simulink model "AERO421_FP7"  (R2024b)
settings: Solver=ode3  StartTime=0.0  StopTime=tspan  FixedStep=5  RelTol=1e-3
values from neighbouring files (symbols this model uses):
  E_b_ECI_0 = C2EulerAngles(C_b_ECI_0)    [AERO421_FP7_RJFSR.m]
  I_s = diag([1.2, 1.2, 1.2])    [AERO421_FP7_RJFSR.m]
  J = J + I_w1 + I_w2 + I_w3    [AERO421_FP7_RJFSR.m]
  JD_0 = 2460390    [AERO421_FP7_RJFSR.m]
  Kd = J*eye(3)*2*zeta*wn    [AERO421_FP7_RJFSR.m]
  Kp = 2*J*eye(3)*wn^2    [AERO421_FP7_RJFSR.m]
  m_b = [0; 0; -0.5]    [AERO421_FP7_RJFSR.m]
  max_T = 1    [AERO421_FP7_RJFSR.m]
  q_b_ECI_0 = rotm2quat(C_b_ECI_0)    [AERO421_FP7_RJFSR.m]
  sun_ECI = [0 0 -1]    [AERO421_FP7_RJFSR.m]
  surfaceProperties = [Areas cps normals ... (first row only)    [AERO421_FP7_RJFSR.m]
  w_b_ECI_0 = [0.001; -0.001; 0.002]    [AERO421_FP7_RJFSR.m]
undefined symbols (not defined in the file or in its folder): r_ECI_0, v_ECI_0
libraries: aerolibutil x1
settings Model: Creator=rosha  LastModifiedBy=rosha

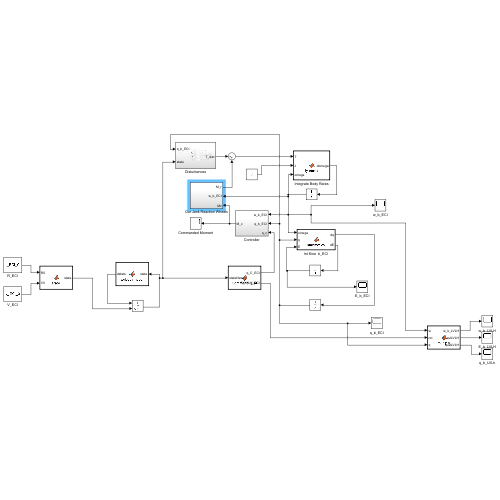
[thumbnail: Simulink's stored preview of the top-level diagram]
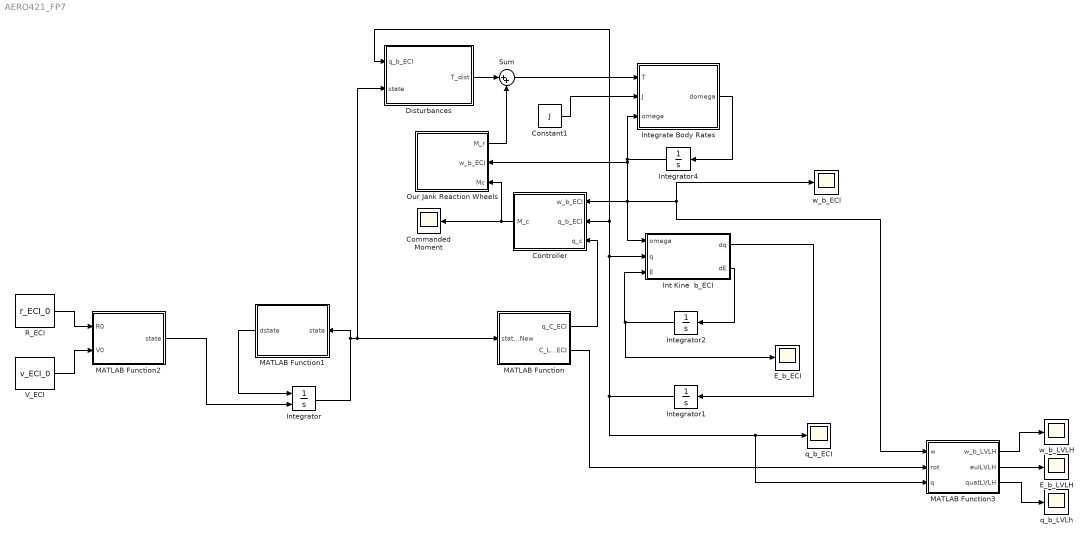
== system AERO421_FP7 ==
  Commanded Moment : Scope
  Constant1 : Constant  Value=J
  Controller : Subsystem
  Disturbances : Subsystem
  E_b_ECI : Scope
  E_b_LVLH : Scope
  Int Kine  b_ECI : MATLAB Function  TreatAsAtomicUnit=on
  Integrate Body Rates : MATLAB Function  TreatAsAtomicUnit=on
  Integrator : Integrator  InitialConditionSource=external
  Integrator1 : Integrator  InitialCondition=q_b_ECI_0
  Integrator2 : Integrator  InitialCondition=E_b_ECI_0
  Integrator4 : Integrator  InitialCondition=w_b_ECI_0
  MATLAB Function : MATLAB Function  TreatAsAtomicUnit=on
  MATLAB Function1 : MATLAB Function  TreatAsAtomicUnit=on
  MATLAB Function2 : MATLAB Function  TreatAsAtomicUnit=on
  MATLAB Function3 : MATLAB Function  TreatAsAtomicUnit=on
  Our Jank Reaction Wheels : Subsystem
      settings: PortSchema="{\"entries\":[{\"content\":{\"sides\":[{\"content\":{\"connectorIds\":[\"Out1\",\"In1\",\"In2\"]},\"type\":\"ConnectorPlacement.EquallySpacedRectSide\",\"uuid\":\"c07e65a8-3a09-4163-ab9e-2228d2e52ec5\"},{\"content\":{\"side\":\"RIGHT\"},\"type\":\"ConnectorPlacement.EquallySpacedRectSide\",\"uuid\":\"64fc0568-6df4-40c5-97b1-a675a03b9b7b\"},{\"content\":{\"side\":\"TOP\"},\"type\":\"ConnectorPlacement.EquallySpacedRectSide\",\"uuid\":\"6ced51b5-350f-46bd-bff5-546870cdfb70\"}]},\"type\":\"ConnectorPlacement.EquallySpacedConnector\",\"uuid\":\"a6912720-308f-478a-9475-f02870833daa\"}],\"packageUris\":[\"http://schema.mathworks.com/mf0/Connector/R2020b\"],\"version\":\"1.0\"}"
  R_ECI : Constant  Value=r_ECI_0
  Sum : Sum  Inputs=|++
  V_ECI : Constant  Value=v_ECI_0
  q_b_ECI : Scope
  q_b_LVLh : Scope
  w_b_ECI : Scope
  w_b_LVLH : Scope
  wires:
  Integrator1/1 -> Disturbances/1(q_b_ECI), Controller/2(q_b_ECI), Int Kine  b_ECI/2(q), MATLAB Function3/3(q), q_b_ECI/1
  MATLAB Function3/2(eulLVLH) -> E_b_LVLH/1
  Constant1/1 -> Integrate Body Rates/2(J)
  V_ECI/1 -> MATLAB Function2/2(V0)
  Integrator2/1 -> E_b_ECI/1, Int Kine  b_ECI/3(E)
  MATLAB Function3/1(w_b_LVLH) -> w_b_LVLH/1
  MATLAB Function/1(q_C_ECI) -> Controller/3(q_c)
  MATLAB Function2/1(state) -> Integrator/2
  MATLAB Function/2(C_LVLH_ECI) -> MATLAB Function3/2(rot)
  Int Kine  b_ECI/2(dE) -> Integrator2/1
  Controller/1(M_c) -> Commanded Moment/1, Our Jank Reaction Wheels/2(Mc)
  Our Jank Reaction Wheels/1(M_r) -> Sum/2
  Integrate Body Rates/1(domega) -> Integrator4/1
  Int Kine  b_ECI/1(dq) -> Integrator1/1
  Integrator4/1 -> Our Jank Reaction Wheels/1(w_b_ECI), MATLAB Function3/1(w), w_b_ECI/1, Int Kine  b_ECI/1(omega), Controller/1(w_b_ECI), Integrate Body Rates/3(omega)
  R_ECI/1 -> MATLAB Function2/1(R0)
  MATLAB Function1/1(dstate) -> Integrator/1
  MATLAB Function3/3(quatLVLH) -> q_b_LVLh/1
  Integrator/1 -> Disturbances/2(state), MATLAB Function/1(stateNew), MATLAB Function1/1(state)
  Disturbances/1(T_dist) -> Sum/1
  Sum/1 -> Integrate Body Rates/1(T)

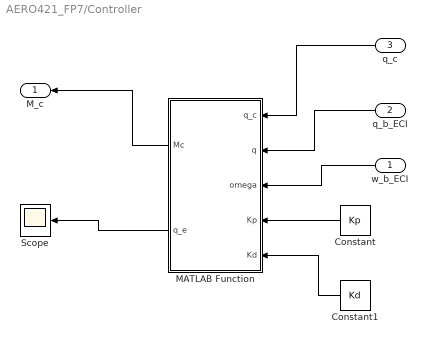
== system AERO421_FP7/Controller ==
  w_b_ECI : Inport  PortDimensions=[3 1]
  q_b_ECI : Inport  Port=2  PortDimensions=[4 1]
  q_c : Inport  Port=3  PortDimensions=[4 1]
  Constant : Constant  Value=Kp
  Constant1 : Constant  Value=Kd
  MATLAB Function : MATLAB Function  TreatAsAtomicUnit=on
  Scope : Scope
  M_c : Outport  PortDimensions=[3 1]  VectorParamsAs1DForOutWhenUnconnected=off
  wires:
  MATLAB Function/1(Mc) -> M_c/1
  q_c/1 -> MATLAB Function/1(q_c)
  q_b_ECI/1 -> MATLAB Function/2(q)
  w_b_ECI/1 -> MATLAB Function/3(omega)
  Constant/1 -> MATLAB Function/4(Kp)
  Constant1/1 -> MATLAB Function/5(Kd)
  MATLAB Function/2(q_e) -> Scope/1

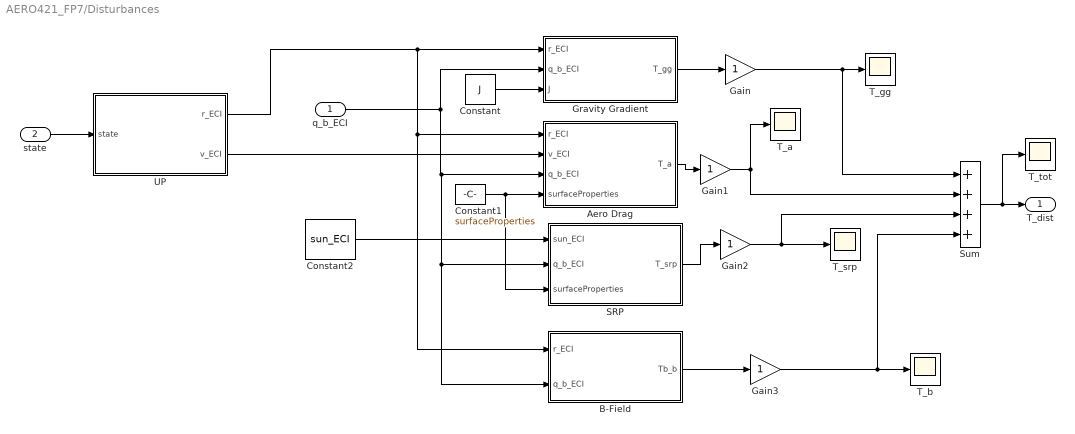
== system AERO421_FP7/Disturbances ==
  q_b_ECI : Inport
  state : Inport  Port=2
  Aero Drag : MATLAB Function  TreatAsAtomicUnit=on
  B-Field : Subsystem
  Constant : Constant  Value=J
  Constant1 : Constant  Value=surfaceProperties
  Constant2 : Constant  Value=sun_ECI
  Gain{,1..3} (4 alike) : Gain
  Gravity Gradient : MATLAB Function  TreatAsAtomicUnit=on
  SRP : MATLAB Function  TreatAsAtomicUnit=on
  Sum : Sum  Inputs=++++
  T_a : Scope
  T_b : Scope
  T_gg : Scope
  T_srp : Scope
  T_tot : Scope
  UP : MATLAB Function  TreatAsAtomicUnit=on
  T_dist : Outport
  wires:
  Sum/1 -> T_tot/1, T_dist/1
  Aero Drag/1(T_a) -> Gain1/1
  Gravity Gradient/1(T_gg) -> Gain/1
  SRP/1(T_srp) -> Gain2/1
  Constant1/1 -> SRP/3(surfaceProperties), Aero Drag/4(surfaceProperties)
  UP/2(v_ECI) -> Aero Drag/2(v_ECI)
  q_b_ECI/1 -> B-Field/2(q_b_ECI), SRP/2(q_b_ECI), Aero Drag/3(q_b_ECI), Gravity Gradient/2(q_b_ECI)
  Constant/1 -> Gravity Gradient/3(J)
  Constant2/1 -> SRP/1(sun_ECI)
  UP/1(r_ECI) -> B-Field/1(r_ECI), Aero Drag/1(r_ECI), Gravity Gradient/1(r_ECI)
  B-Field/1(Tb_b) -> Gain3/1
  Gain/1 -> Sum/1, T_gg/1
  Gain1/1 -> Sum/2, T_a/1
  Gain2/1 -> Sum/3, T_srp/1
  Gain3/1 -> T_b/1, Sum/4
  state/1 -> UP/1(state)

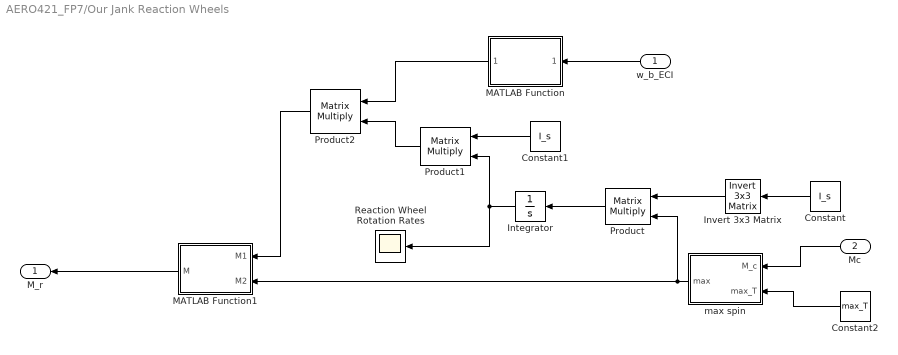
== system AERO421_FP7/Our Jank Reaction Wheels ==
  w_b_ECI : Inport  PortDimensions=[3 1]
  Mc : Inport  Port=2
  Constant : Constant  Value=I_s
  Constant1 : Constant  Value=I_s
  Constant2 : Constant  Value=max_T
  Integrator : Integrator
  Invert 3x3 Matrix : aerolibutil/Invert  3x3 Matrix
  MATLAB Function : MATLAB Function  TreatAsAtomicUnit=on
  MATLAB Function1 : MATLAB Function  TreatAsAtomicUnit=on
  Product : Product  Multiplication=Matrix(*)
  Product1 : Product  Multiplication=Matrix(*)
  Product2 : Product  Multiplication=Matrix(*)
  Reaction Wheel Rotation Rates : Scope
  max spin : MATLAB Function  TreatAsAtomicUnit=on
  M_r : Outport  PortDimensions=[3 1]  VectorParamsAs1DForOutWhenUnconnected=off
  wires:
  MATLAB Function1/1(M) -> M_r/1
  w_b_ECI/1 -> MATLAB Function/1(omega)
  Invert 3x3 Matrix/1 -> Product/1
  Constant/1 -> Invert 3x3 Matrix/1
  Product/1 -> Integrator/1
  Integrator/1 -> Reaction Wheel Rotation Rates/1, Product1/2
  Constant1/1 -> Product1/1
  Product2/1 -> MATLAB Function1/1(M1)
  Product1/1 -> Product2/2
  MATLAB Function/1(omegaX) -> Product2/1
  max spin/1(max) -> Product/2, MATLAB Function1/2(M2)
  Mc/1 -> max spin/1(M_c)
  Constant2/1 -> max spin/2(max_T)

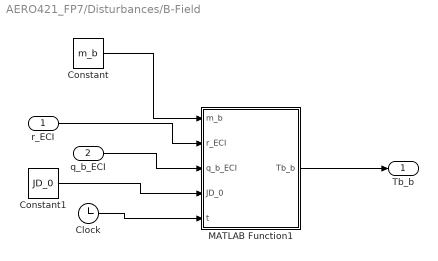
== system AERO421_FP7/Disturbances/B-Field ==
  r_ECI : Inport
  q_b_ECI : Inport  Port=2
  Clock : Clock
  Constant : Constant  Value=m_b  VectorParams1D=off
  Constant1 : Constant  Value=JD_0
  MATLAB Function1 : MATLAB Function  TreatAsAtomicUnit=on
  Tb_b : Outport
  wires:
  MATLAB Function1/1(Tb_b) -> Tb_b/1
  q_b_ECI/1 -> MATLAB Function1/3(q_b_ECI)
  r_ECI/1 -> MATLAB Function1/2(r_ECI)
  Clock/1 -> MATLAB Function1/5(t)
  Constant1/1 -> MATLAB Function1/4(JD_0)
  Constant/1 -> MATLAB Function1/1(m_b)

== matlab function AERO421_FP7/Disturbances/Gravity Gradient ==
  data: r_ECI input; T_gg output; q_b_ECI input; J input
function T_gg = gg_torque(r_ECI, q_b_ECI, J)
mu = 398600; % km^3/s^2

C_b_ECI = quat2dcm(q_b_ECI');
r_b = C_b_ECI * r_ECI;

T_gg = 3*mu/norm(r_ECI)^5*vcross(r_b)*J*r_b;

end

== matlab function AERO421_FP7/Controller/MATLAB Function ==
  data: q_c input; Mc output; q input; omega input; Kp input; Kd input; q_e output
function [Mc,q_e]  = control_law(q_c, q, omega, Kp, Kd)
%#codegen

%q_e = quatMult(quatConjugate(q_c), q);
q_e = quatMult(q, quatConjugate(q_c));
Mc = -Kp*q_e(1:3,1) - Kd*omega;

== matlab function AERO421_FP7/Disturbances/SRP ==
  data: sun_ECI input; T_srp output; q_b_ECI input; surfaceProperties input
function T_srp  = SPR_torque(sun_ECI, q_b_ECI, surfaceProperties)

p_sun = 4.5e-6; %N/m (given)
C_b_ECI_0 = quat2dcm(q_b_ECI');
sun_b = C_b_ECI_0*sun_ECI;
sun_hat = sun_b/norm(sun_b);
T_srp = [0; 0; 0];

for i = 1:length(surfaceProperties)
    % Find wetted area
    normVect = surfaceProperties(i, 5:7);
    normVect = normVect/norm(normVect);
    cpa = surfaceProperties(i, 2:4);
    areaSurf = surfaceProperties(i, 1);
    A_wet = areaSurf*dot(normVect, sun_hat);
    if A_wet > 0
        % Add to total torque from solar pressure
        F_sun = -p_sun*sun_hat*A_wet;
        T_srp = T_srp + cross(cpa', F_sun);
    end
end
end

== matlab function AERO421_FP7/Disturbances/UP ==
  data: state input; r_ECI output; v_ECI output
function [r_ECI, v_ECI]  = unpack(state)

r_ECI = state(1:3)';
v_ECI = state(4:6)';

== matlab function AERO421_FP7/Our Jank Reaction Wheels/max spin ==
  data: M_c input; max output; max_T input
function max = maxT(M_c,max_T)

if norm(M_c) <= max_T
    max = M_c;
else
    max = max_T * M_c/norm(M_c);
end

== matlab function AERO421_FP7/Our Jank Reaction Wheels/MATLAB Function1 ==
  data: M1 input; M output; M2 input
function M = matAdd(M1, M2)
M = M1 + M2;

== matlab function AERO421_FP7/Our Jank Reaction Wheels/MATLAB Function ==
  data: omega input; omegaX output
function omegaX = omegaCross(omega)
omegaX = vcross(omega);

== matlab function AERO421_FP7/MATLAB Function ==
  data: stateNew input; q_C_ECI output; C_LVLH_ECI output
function [q_C_ECI,C_LVLH_ECI] = CommandQuat(stateNew)

R = [stateNew(end,1); stateNew(end,2); stateNew(end,3)];
V = [stateNew(end,4); stateNew(end,5); stateNew(end,6)];

R = R'; %in ECI
V = V';

Z_lvlh = -R/norm(R);
Y_lvlh = -cross(R,V)/norm(cross(R,V));
X_lvlh = cross(Y_lvlh,Z_lvlh);

C_LVLH_ECI = [X_lvlh',Y_lvlh',Z_lvlh'];
C_ECI_LVLH = C_LVLH_ECI';

pointingLVLH = [0;0;-1]; %pointing nadir (always at ground station)

eul = C_ECI_LVLH*pointingLVLH;

q = eul2quat(eul')';
n = q(1);
e = q(2:4);

q_C_ECI = [e;n];

== matlab function AERO421_FP7/MATLAB Function1 ==
  data: state input; dstate output
function dstate = twobodymotion(state) %dstate is derivitve of state
%FUNCTION put in descrip    

mu = 398600;

    %define vars
    x = state(1);
    y = state(2);
    z = state(3);
    dx = state(4); %vel
    dy = state(5); %vel
    dz = state(6); %vel
    
    %mag of pos vector
    r = norm([x y z]);
    
    %accel: !!eqs of motion!!
    ddx = -mu*x/r^3;
    ddy = -mu*y/r^3;
    ddz = -mu*z/r^3;
    
    dstate = [dx; dy; dz; ddx; ddy; ddz]';

end

== matlab function AERO421_FP7/Int Kine  b_ECI ==
  data: omega input; q input; dq output; E input; dE output
function [dq,dE] = kinematics(omega, q, E)
%#codegen

% unpack quaternion

epsilon = q(1:3,1);
eta = q(4,1);

depsilon = 1/2*(eta*eye(3) + vcross(epsilon))*omega;
deta = -1/2*epsilon'*omega;

dq = [depsilon; deta];

LBI = 1/cos(E(2))*[cos(E(2)) sin(E(1))*sin(E(2))  cos(E(1))*sin(E(2));
                   0         cos(E(1))*cos(E(2)) -sin(E(1))*cos(E(2));
                   0         sin(E(1))            cos(E(1))];

dE = LBI*omega;

== matlab function AERO421_FP7/Integrate Body Rates ==
  data: T input; J input; omega input; domega output
function domega = dynamics(T, J, omega)
%#codegen

domega = J\(T - cross(omega, J*omega));

== matlab function AERO421_FP7/MATLAB Function2 ==
  data: R0 input; state output; V0 input
function state = state(R0,V0)

state = [R0',V0'];

== matlab function AERO421_FP7/MATLAB Function3 ==
  data: w input; rot input; w_b_LVLH output; q input; eulLVLH output; quatLVLH output
function [w_b_LVLH,eulLVLH,quatLVLH] = multiply(w,rot,q)

w_b_LVLH = rot*w;

n = q(4);
e = q(1:3)';
quat = [n,e];
eul = quat2eul(quat);

eulLVLH = rot*eul';

q2 = eul2quat(eulLVLH')';
n = q2(1);
e = q2(2:4);
quatLVLH = [e;n];

== matlab function AERO421_FP7/Disturbances/Aero Drag ==
  data: r_ECI input; v_ECI input; T_a output; q_b_ECI input; surfaceProperties input
function T_a = aero_drag_torque(r_ECI, v_ECI, q_b_ECI, surfaceProperties) 
r_ECI = r_ECI*1000; % m
v_ECI = v_ECI*1000; % m/s
% Convert v_ECI to v_b
C_b_ECI_0 = quat2dcm(q_b_ECI');
v_b = C_b_ECI_0*v_ECI;
v_hat = v_b/norm(v_b);
% Calculate density using standard exponetial decay model (or model of your
% choice)
Re = 6378*1000;
Me = 5.972e+24;
h = norm(r_ECI) - Re;
G = 6.67e-11;
k = 1.381e-23;
rho0 = 3.614e-14;
Cd = 2.2;

g = G*Me/norm(r_ECI)^2;

m = 28.964/6.022e23; % CHECK UNITS
T = - 131.21 + 0.00299*h;
H = 109*1000;
h0 = 700*1000;
rho = rho0*exp(-((h-h0)/H));
T_a = [0; 0; 0];
% P = 22.65 * exp(1.73 - .000157 * h);
% rho = P/(0.2869*(T+273.15));



% Loop through all the surfaces of the MehielSat
for i = 1:length(surfaceProperties)
    % Find wetted area
    normVect = surfaceProperties(i, 5:7);
    normVect = normVect/norm(normVect);
    cpa = surfaceProperties(i, 2:4);
    areaSurf = surfaceProperties(i, 1);
    A_wet = areaSurf*dot(normVect, v_hat);
    if A_wet > 0
        % Add to total torque from atmospheric drag
        Fdrag = -0.5*Cd*rho*norm(v_b)^2*A_wet*v_hat;
        T_a = T_a + cross(cpa', Fdrag);
    end


end

== matlab function AERO421_FP7/Disturbances/B-Field/MATLAB Function1 ==
  data: m_b input; r_ECI input; q_b_ECI input; Tb_b output; JD_0 input; t input
function Tb_b = WMM(m_b, r_ECI, q_b_ECI, JD_0, t)

% Constants
omega_Earth = 7.2921150e-5; % Earth's rotation rate in rad/s
r_ECI = r_ECI*1000; %convert to meters

% Time since JD_0 (in days)
delta_JD = t / 86400; % 86400 sec/day

% Current Julian Date
JD = JD_0 + delta_JD;
pos = omega_Earth*JD;
r_ECEF = rotz(rad2deg(pos))' * r_ECI;

C_b_ECI = quat2dcm(q_b_ECI');
C_ECI_ECEF = rotz(rad2deg(pos));
C_b_ECEF = C_b_ECI * C_ECI_ECEF;

% DGRF 2020 (given)
a = 6371.2; %km
g_11 = -1450.9; %nT
h_11 = 4652.5; %nT
g_10 = -29404.8; %nT
m_ECEF = a^3*[g_11; h_11; g_10]; %nT km^3
m_ECEF = m_ECEF * 1e-9 * (1e3)^3; % convert nT to T, km^3 to m^3


m = m_ECEF;
r = r_ECEF;
B = (3*dot(m,r)*r - m*norm(r)^2) / norm(r)^5; %in ECEF
B_b = C_b_ECEF * B;

Tb_b = cross(m_b,B_b);
